simulink model "Monza_controlado"  (R2021b)
settings: Solver=VariableStepAuto  StartTime=0.0  StopTime=20  FixedStep=Ts  RelTol=1e-3
StopFcn:
  | %animacion_monza(dificultad, Ts, giro_m, xs, ys)
values from neighbouring files (symbols this model uses):
  dificultad = 2    [Modelo.m]    (also in Simulation.m = 1)
undefined symbols (not defined in the file or in its folder): FailDetector
libraries: rllib x1
settings Model: Creator=christian  LastModifiedBy=Guillermo
settings SolverCC: AlgebraicLoopSolver=TrustRegion
settings DataIOCC: ReturnWorkspaceOutputs=off
settings DebuggingCC: SFMachineParentedDataDiag=warning  ArithmeticOperatorsInVariantConditions=warning
settings SFSimCC: SimUseLocalCustomCode=off  CustomCodeUndefinedFunction=UseInterfaceOnly
settings RTWCC: RTWUseLocalCustomCode=off

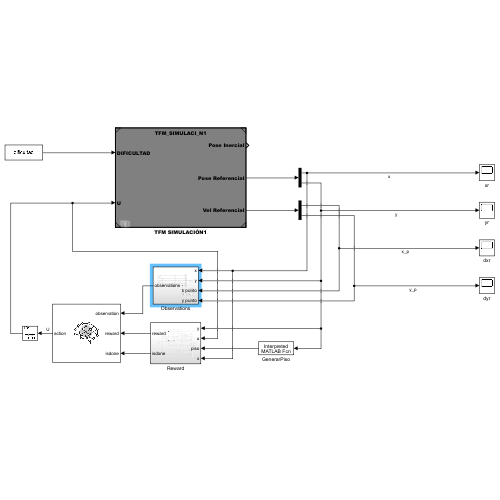
[thumbnail: Simulink's stored preview of the top-level diagram]
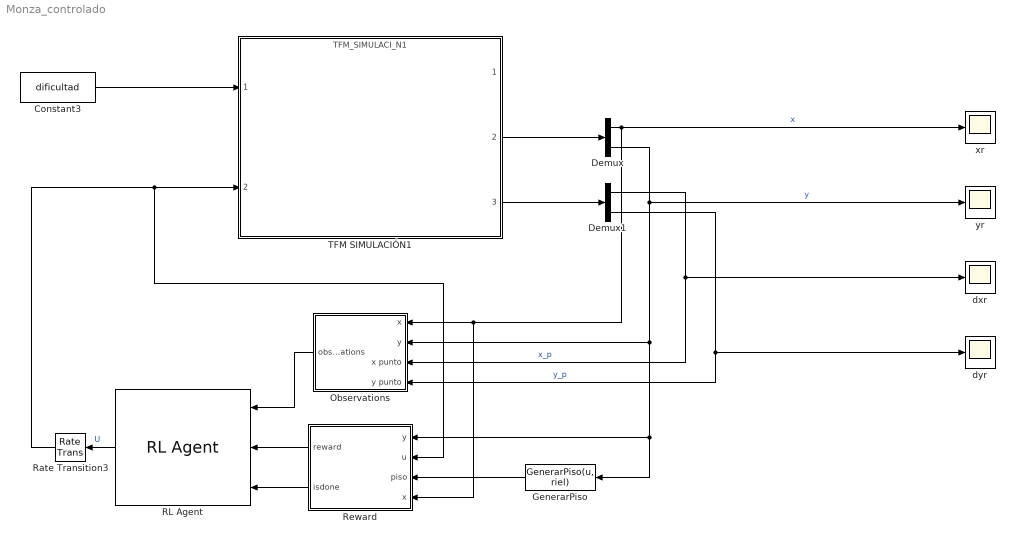
== system Monza_controlado ==
  Constant3 : Constant  Value=dificultad
  Demux : Demux  Outputs=2
  Demux1 : Demux  Outputs=2
  GenerarPiso : MATLABFcn  MATLABFcn=GenerarPiso(u, riel)
  Observations : Subsystem
  RL Agent : rllib/RL Agent  Agent=agent1_Trained  ExternalActionAsInput=off  ProvideCumRwd=off  TreatAsDirectFeedthrough=on
  Rate Transition3 : RateTransition  OutPortSampleTime=0
  Reward : Subsystem
  TFM SIMULACIÓN1 : ModelReference  ModelNameDialog=TFM_SIMULACI_N1.slx  UsingDefaultArgumentValue=0,0  SimulationMode=Normal  ModelReferenceVersion=9.19  Gain=0.05  Gain2=0.0223  SimulationMode=Normal
  dxr : Scope
  dyr : Scope
  xr : Scope
  yr : Scope
  wires:
  Constant3/1 -> TFM SIMULACIÓN1/1
  TFM SIMULACIÓN1/2 -> Demux/1
  TFM SIMULACIÓN1/3 -> Demux1/1
  Demux1/1 -> Observations/3(x punto), dxr/1  "x_p"
  Demux/1 -> xr/1, Reward/4(x), Observations/1(x)  "x"
  Demux/2 -> Observations/2(y), GenerarPiso/1, Reward/1(y), yr/1  "y"
  Demux1/2 -> dyr/1, Observations/4(y punto)  "y_p"
  RL Agent/1 -> Rate Transition3/1  "U"
  Reward/1(reward) -> RL Agent/2
  Observations/1(observations) -> RL Agent/1
  Reward/2(isdone) -> RL Agent/3
  GenerarPiso/1 -> Reward/3(piso)
  Rate Transition3/1 -> Reward/2(u), TFM SIMULACIÓN1/2

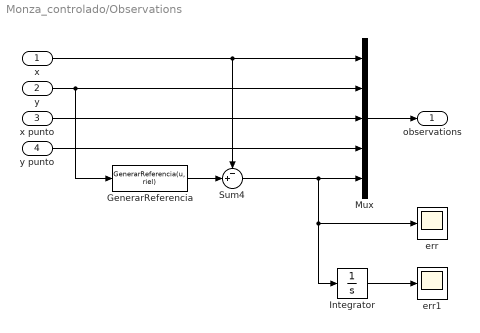
== system Monza_controlado/Observations ==
  x : Inport
  y : Inport  Port=2
  x punto : Inport  Port=3
  y punto : Inport  Port=4
  GenerarReferencia : MATLABFcn  MATLABFcn=GenerarReferencia(u, riel)
  Integrator : Integrator
  Mux : Mux  Inputs=5
  Sum4 : Sum  Inputs=-+|
  err : Scope
  err1 : Scope
  observations : Outport
  wires:
  y/1 -> GenerarReferencia/1, Mux/2
  y punto/1 -> Mux/4
  x/1 -> Mux/1, Sum4/1
  Mux/1 -> observations/1
  x punto/1 -> Mux/3
  GenerarReferencia/1 -> Sum4/2
  Sum4/1 -> Integrator/1, err/1, Mux/5
  Integrator/1 -> err1/1

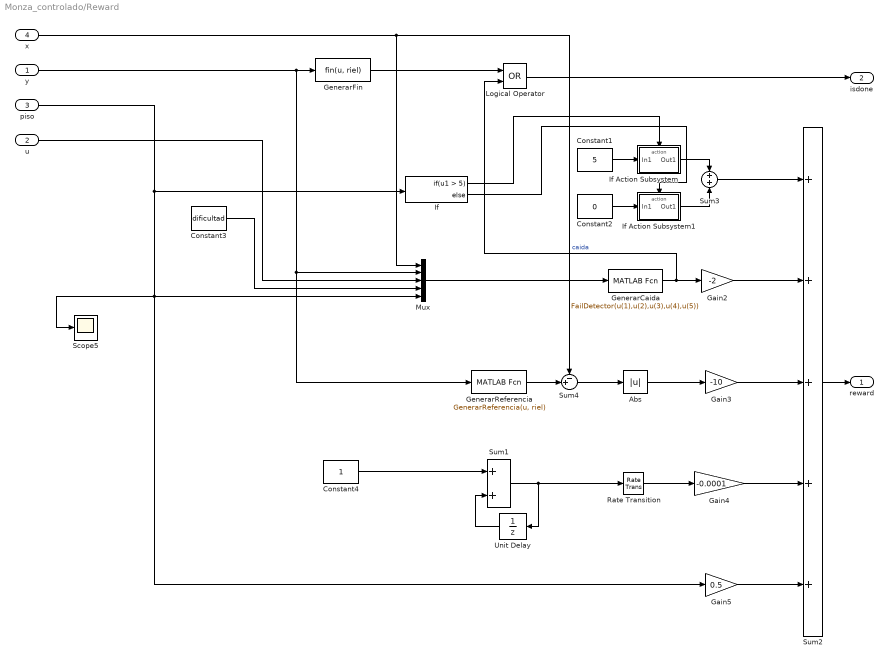
== system Monza_controlado/Reward ==
  y : Inport
  u : Inport  Port=2
  piso : Inport  Port=3
  x : Inport  Port=4
  Abs : Abs
  Constant1 : Constant  Value=5
  Constant2 : Constant  Value=0
  Constant3 : Constant  Value=dificultad
  Constant4 : Constant
  Gain2 : Gain  Gain=-2
  Gain3 : Gain  Gain=-10
  Gain4 : Gain  Gain=-0.0001
  Gain5 : Gain  Gain=0.5
  GenerarCaida : MATLABFcn  MATLABFcn=FailDetector(u(1),u(2),u(3),u(4),u(5))  OutputDimensions=1
  GenerarFin : MATLABFcn  MATLABFcn=fin(u, riel)  OutputDimensions=1
  GenerarReferencia : MATLABFcn  MATLABFcn=GenerarReferencia(u, riel)
  If : If  IfExpression=u1 > 5
  If Action Subsystem : Subsystem  TreatAsAtomicUnit=on
  If Action Subsystem1 : Subsystem  TreatAsAtomicUnit=on
  Logical Operator : Logic  Operator=OR  AllPortsSameDT=off  OutDataTypeStr=boolean
  Mux : Mux  Inputs=5
  Rate Transition : RateTransition  OutPortSampleTime=Ts
  Scope5 : Scope
  Sum1 : Sum
  Sum2 : Sum  Inputs=+++++
  Sum3 : Sum
  Sum4 : Sum  Inputs=-+|
  Unit Delay : UnitDelay  SampleTime=-1  HasFrameUpgradeWarning=on
  reward : Outport  VectorParamsAs1DForOutWhenUnconnected=off
  isdone : Outport  Port=2  VectorParamsAs1DForOutWhenUnconnected=off
  wires:
  y/1 -> GenerarReferencia/1, Mux/2, GenerarFin/1
  Sum2/1 -> reward/1
  GenerarCaida/1 -> Logical Operator/2, Gain2/1  "caida"
  Gain2/1 -> Sum2/2
  GenerarFin/1 -> Logical Operator/1
  Logical Operator/1 -> isdone/1
  Constant3/1 -> Mux/4
  Mux/1 -> GenerarCaida/1
  u/1 -> Mux/3
  piso/1 -> Gain5/1, Mux/5, Scope5/1, If/1
  If/1 -> If Action Subsystem/Action
  Constant1/1 -> If Action Subsystem/1(In1)
  If/2 -> If Action Subsystem1/Action
  Constant2/1 -> If Action Subsystem1/1(In1)
  Sum3/1 -> Sum2/1
  If Action Subsystem/1(Out1) -> Sum3/1
  If Action Subsystem1/1(Out1) -> Sum3/2
  x/1 -> Sum4/1, Mux/1
  Rate Transition/1 -> Gain4/1
  Sum1/1 -> Unit Delay/1, Rate Transition/1
  Gain4/1 -> Sum2/4
  Constant4/1 -> Sum1/1
  Unit Delay/1 -> Sum1/2
  Gain5/1 -> Sum2/5
  GenerarReferencia/1 -> Sum4/2
  Gain3/1 -> Sum2/3
  Sum4/1 -> Abs/1
  Abs/1 -> Gain3/1

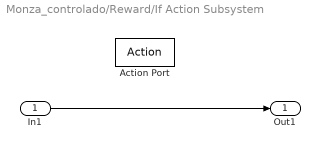
== system Monza_controlado/Reward/If Action Subsystem ==
  In1 : Inport
  Action Port : ActionPort  ActionPortLabel=if(u1 > 5)
  Out1 : Outport
  wires:
  In1/1 -> Out1/1

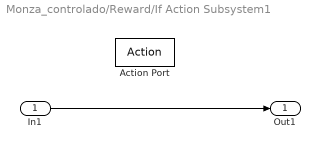
== system Monza_controlado/Reward/If Action Subsystem1 ==
  In1 : Inport
  Action Port : ActionPort  ActionPortLabel=else
  Out1 : Outport
  wires:
  In1/1 -> Out1/1
